simulink model "RL_TTS3_Controller_Blank"  (R2019b)
settings: Solver=FixedStepAuto  StartTime=0.0  StopTime=10.0  FixedStep=0.01  RelTol=1e-3
PostLoadFcn:
  | if any(exist('dsrtsu_mdlpostloadfcn', 'file') ~= 0), dsrtsu_mdlpostloadfcn('Execute', bdroot); end
libraries: simulink x1
settings Model: DSRTSU_INTERNAL_RTI_VER=550  DSRTSU_INTERNAL_RTI_TYPE=rti1104  RTICANMMDATA=struct('GeneralSetupData',struct('modelroot','E:\Will\RemoteLabs\TTS3\HostPC','generalsettings',struct('filesettings',struct('destfolder',struct('Name','RTICANMM_FILES','Check',1),'buildfolder',struct('Name','.','Check',1),'AbsDestfolder',struct('Name','E:\Will\RemoteLabs\TTS3\HostPC\RTICANMM_FILES'),'AbsBuildfolder',struct('Name','E:\Will\RemoteLabs\TTS3\HostPC'))),'options',struct('addpaths',1,'rmpaths',1,'addtrcexclusion',true,'cannavigator',struct('checkmonitoring',0),'show_usrtrc',0,'use_usrtrc',0),'advanced',struct('options',ones(1,100)),'MPSetup',{{}},'RTI',struct('Type','RTI1104','Ver','7.13','Date','02-Nov-2019'),'modelname','TTS3_Controller_Test_OL','block','TTS3_Controller_Test_OL'))  DSRTSU_INTERNAL_RTIFPGA=150  Creator=whendrix  LastModifiedBy=edtve
settings OptimizationCC: BlockReduction=off  DefaultParameterBehavior=Inlined  OptimizeBlockIOStorage=off  BufferReuse=off  GlobalBufferReuse=off  ExpressionFolding=off  LocalBlockOutputs=off  OptimizeDataStoreBuffers=off  BusAssignmentInplaceUpdate=off
settings DebuggingCC: BusObjectLabelMismatch=none
settings HardwareCC: ProdBitPerPointer=32  ProdBitPerSizeT=32  ProdBitPerPtrDiffT=32  ProdLargestAtomicInteger=Integer  ProdEndianess=BigEndian  ProdWordSize=32  ProdHWDeviceType=Custom Processor->Custom  TargetIntDivRoundTo=Zero  TargetEndianess=BigEndian  TargetHWDeviceType=Custom Processor->Custom
settings ModelReferenceCC: ModelReferenceNumInstancesAllowed=Single  ModelReferenceMinAlgLoopOccurrences=on
settings SFSimCC: MATLABDynamicMemAlloc=off  CustomCodeUndefinedFunction=UseInterfaceOnly
settings RTWCC: Description=dSPACE DS1104 Hardware Platform  SystemTargetFile=rti1104.tlc  MakeCommand=make_rti  TemplateMakefile=rti1104.tmf
settings CodeAppCC: MaxIdLength=63
settings STFCustomTargetCC: ParMdlRefBuildCompliant=on  SystemTargetFile=rti1104.tlc
settings GRTTargetCC: TargetLangStandard=C89/C90 (ANSI)  CompOptLevelCompliant=off  ConcurrentExecutionCompliant=off  CombineOutputUpdateFcns=off  MatFileLogging=off  CPPClassGenCompliant=off  UseToolchainInfoCompliant=off

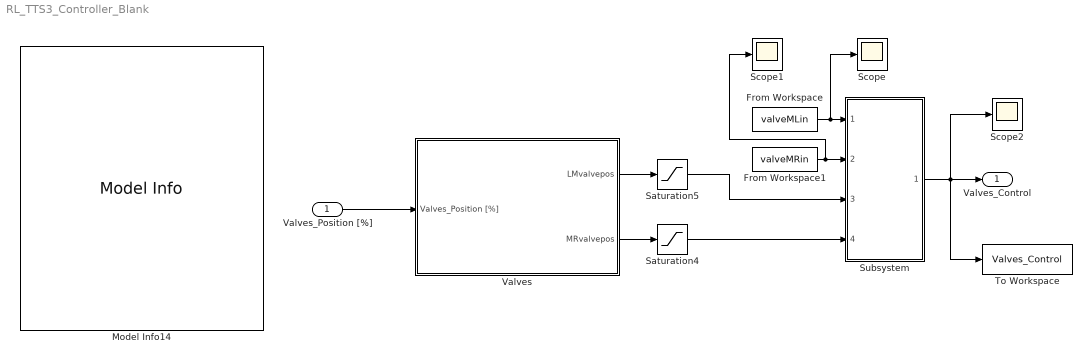
== system RL_TTS3_Controller_Blank ==
  Valves_Position [%] : Inport  OutDataTypeStr=Bus: ValvesSOCI
  From Workspace : FromWorkspace  VariableName=valveMLin  SampleTime=0
  From Workspace1 : FromWorkspace  VariableName=valveMRin  SampleTime=0
  Model Info14 : simulink/Model-Wide Utilities/Model Info  Frame=on  DisplayStringWithTags=|  HorizontalTextAlignment=Left  LeftAlignmentValue=0.02
      | Start model for the "Three Tank"
      | experiment on the "Three Tank" setup.
      | Version: 1.0
      | 
      | 
      | INFORMATION
      | ----------------------
      | 
      | Unity Gain block before Scope is needed for
      | RemoteLabs compatebility. 
      | Do not modify or remove!
      | 
      | Pump range:
      | 0 to 0.102 [l/s]
      | 
      | The 5 Valves are labeled according 
      | to their position:
      | 
      |    LM  MR
      |      X     X
      |  X      X      X
      | LD    MD   RD
      | 
      | L = Left
      | M = Middle
      | R = Right
      | D = Down
  Saturation4 : Saturate  UpperLimit=100  LowerLimit=0
  Saturation5 : Saturate  UpperLimit=100  LowerLimit=0
  Scope : Scope
  Scope1 : Scope
  Scope2 : Scope
  Subsystem : Subsystem
  To Workspace : ToWorkspace  VariableName=Valves_Control  SaveFormat=Timeseries  SampleTime=-1
  Valves : Subsystem  TreatAsAtomicUnit=on
  Valves_Control : Outport  OutDataTypeStr=Bus: ValvesSICO  VectorParamsAs1DForOutWhenUnconnected=off
  wires:
  Valves_Position [%]/1 -> Valves/1(Valves_Position [%])
  Subsystem/1(Valves1) -> To Workspace/1, Scope2/1, Valves_Control/1
  Valves/1(LMvalvepos) -> Saturation5/1
  Valves/2("MRvalvepos ") -> Saturation4/1
  Saturation5/1 -> Subsystem/3(MLValvepos)
  From Workspace/1 -> Scope/1, Subsystem/1("MLValveOpen ")
  From Workspace1/1 -> Scope1/1, Subsystem/2(MRvalveOpen)
  Saturation4/1 -> Subsystem/4(MRValvepos)

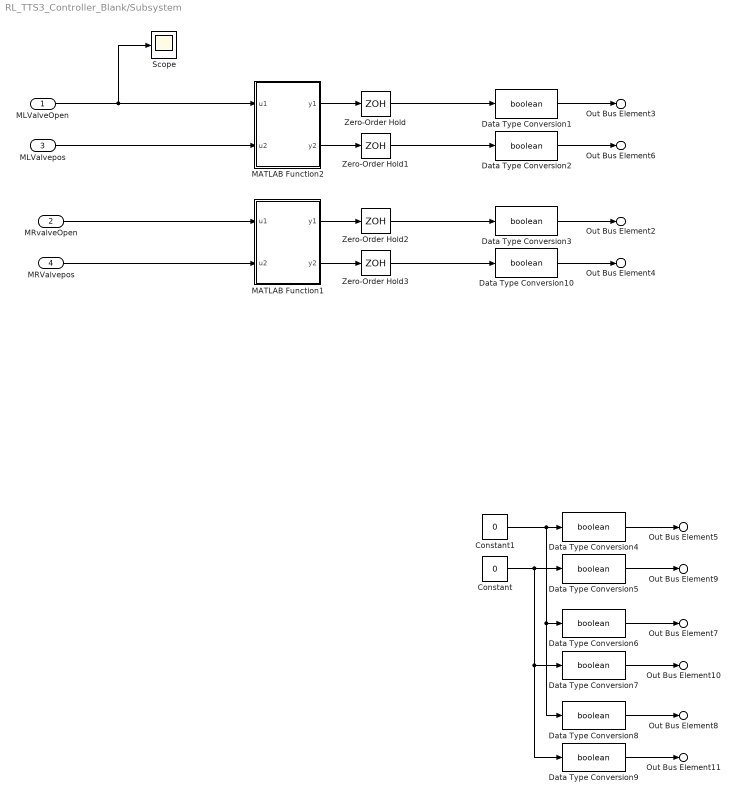
== system RL_TTS3_Controller_Blank/Subsystem ==
  "MLValveOpen " : Inport
  MRvalveOpen : Inport  Port=2
  MLValvepos : Inport  Port=3
  MRValvepos : Inport  Port=4
  Constant : Constant  Value=0
  Constant1 : Constant  Value=0
  Data Type Conversion{1..10} (10 alike) : DataTypeConversion  OutDataTypeStr=boolean
  MATLAB Function1 : MATLAB Function  TreatAsAtomicUnit=on
  MATLAB Function2 : MATLAB Function  TreatAsAtomicUnit=on
  Scope : Scope
  Zero-Order Hold{,1..3} (4 alike) : ZeroOrderHold  SampleTime=0.5
  Out Bus Element8 : Outport  VectorParamsAs1DForOutWhenUnconnected=off  PortName=Valves1  Element=RightDown.Open
  Out Bus Element11 : Outport  VectorParamsAs1DForOutWhenUnconnected=off  PortName=Valves1  Element=RightDown.Close
  Out Bus Element5 : Outport  VectorParamsAs1DForOutWhenUnconnected=off  PortName=Valves1  Element=LeftDown.Open
  Out Bus Element9 : Outport  VectorParamsAs1DForOutWhenUnconnected=off  PortName=Valves1  Element=LeftDown.Close
  Out Bus Element7 : Outport  VectorParamsAs1DForOutWhenUnconnected=off  PortName=Valves1  Element=MiddleDown.Open
  Out Bus Element10 : Outport  VectorParamsAs1DForOutWhenUnconnected=off  PortName=Valves1  Element=MiddleDown.Close
  Out Bus Element2 : Outport  VectorParamsAs1DForOutWhenUnconnected=off  PortName=Valves1  Element=MiddleRight.Open
  Out Bus Element4 : Outport  VectorParamsAs1DForOutWhenUnconnected=off  PortName=Valves1  Element=MiddleRight.Close
  Out Bus Element3 : Outport  VectorParamsAs1DForOutWhenUnconnected=off  PortName=Valves1  Element=LeftMiddle.Open
  Out Bus Element6 : Outport  VectorParamsAs1DForOutWhenUnconnected=off  PortName=Valves1  Element=LeftMiddle.Close
  wires:
  Data Type Conversion4/1 -> Out Bus Element5/1
  Data Type Conversion5/1 -> Out Bus Element9/1
  Data Type Conversion8/1 -> Out Bus Element8/1
  Constant1/1 -> Data Type Conversion8/1, Data Type Conversion6/1, Data Type Conversion4/1
  Data Type Conversion9/1 -> Out Bus Element11/1
  Data Type Conversion7/1 -> Out Bus Element10/1
  Data Type Conversion6/1 -> Out Bus Element7/1
  Constant/1 -> Data Type Conversion9/1, Data Type Conversion7/1, Data Type Conversion5/1
  MATLAB Function1/1(y1) -> Zero-Order Hold2/1
  MATLAB Function1/2(y2) -> Zero-Order Hold3/1
  MRvalveOpen/1 -> MATLAB Function1/1(u1)
  MRValvepos/1 -> MATLAB Function1/2(u2)
  "MLValveOpen "/1 -> Scope/1, MATLAB Function2/1(u1)
  MLValvepos/1 -> MATLAB Function2/2(u2)
  Data Type Conversion2/1 -> Out Bus Element6/1
  Data Type Conversion3/1 -> Out Bus Element2/1
  Data Type Conversion10/1 -> Out Bus Element4/1
  Data Type Conversion1/1 -> Out Bus Element3/1
  MATLAB Function2/1(y1) -> Zero-Order Hold/1
  MATLAB Function2/2(y2) -> Zero-Order Hold1/1
  Zero-Order Hold/1 -> Data Type Conversion1/1
  Zero-Order Hold1/1 -> Data Type Conversion2/1
  Zero-Order Hold2/1 -> Data Type Conversion3/1
  Zero-Order Hold3/1 -> Data Type Conversion10/1

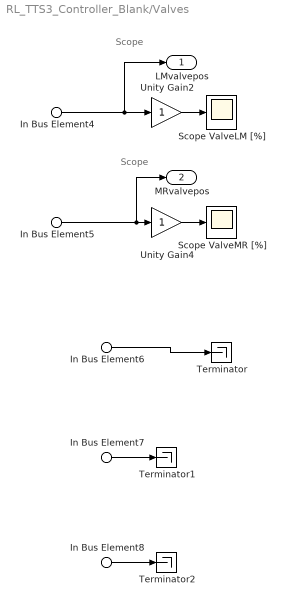
== system RL_TTS3_Controller_Blank/Valves ==
  note: Scope
  note: Scope
  In Bus Element4 : Inport  PortName=Valves_Position [%]  Element=LeftMiddle
  In Bus Element5 : Inport  PortName=Valves_Position [%]  Element=MiddleRight
  In Bus Element6 : Inport  PortName=Valves_Position [%]  Element=LeftDown
  In Bus Element7 : Inport  PortName=Valves_Position [%]  Element=MiddleDown
  In Bus Element8 : Inport  PortName=Valves_Position [%]  Element=RightDown
  Scope ValveLM [%] : Scope
  Scope ValveMR [%] : Scope
  Terminator : Terminator
  Terminator1 : Terminator
  Terminator2 : Terminator
  Unity Gain2 : Gain
  Unity Gain4 : Gain
  LMvalvepos : Outport
  "MRvalvepos " : Outport  Port=2
  wires:
  In Bus Element5/1 -> "MRvalvepos "/1, Unity Gain4/1
  In Bus Element4/1 -> Unity Gain2/1, LMvalvepos/1
  In Bus Element7/1 -> Terminator1/1
  In Bus Element6/1 -> Terminator/1
  In Bus Element8/1 -> Terminator2/1
  Unity Gain4/1 -> Scope ValveMR [%]/1
  Unity Gain2/1 -> Scope ValveLM [%]/1

== matlab function RL_TTS3_Controller_Blank/Subsystem/MATLAB Function2 ==
  data: u1 input; y1 output; y2 output; u2 input
function [y1,y2] = fcn(u1,u2)
    if abs(u1-u2)<=5 % difference is small, set both to false
        y1=false;
        y2 = false;
    elseif u2>u1+5 % position is higher than desired position, set close to true and open to false
        y1 = false;
        y2 = true;
    elseif u1>u2+5 % desired position is higher than position, set open to true and close to false
        y1 = true;
        y2 = false;
    else
        y1 = false;
        y2 = false;
    end
end

== matlab function RL_TTS3_Controller_Blank/Subsystem/MATLAB Function1 ==
  data: u1 input; y1 output; y2 output; u2 input
function [y1,y2] = fcn(u1,u2)
    if abs(u1-u2)<=5
        y1=false;
        y2 = false;
    elseif u2>u1+5
        y1 = false;
        y2 = true;
    elseif u1>u2+5
        y1 = true;
        y2 = false;
    else
        y1 = false;
        y2 = false;
    end
end
